simulink model "VTOL_Y4_Tiltrotor_Model"  (R2015a)
settings: Solver=ode45  StartTime=0.0  StopTime=400  RelTol=1e-3
model workspace (MAT data in the model file):
  op_trim2 : opcond.OperatingReport (value not decoded)
undefined symbols (not defined in the file): sigbuilder_block
libraries: simulink x8, aerolibutil x4, aerolibasang x2, aerolib6dof2 x1, aerolibadyn x1, aerolibconvert2 x1, aerolibtransform2 x1
settings Model: Creator=Swapneel Naphade  LastModifiedBy=HP
settings SolverCC: ZeroCrossControl=DisableAll  ZeroCrossAlgorithm=Adaptive
settings DataIOCC: ExternalInput=getinputstruct(op_trim2)  InitialState=getstatestruct(op_trim2)

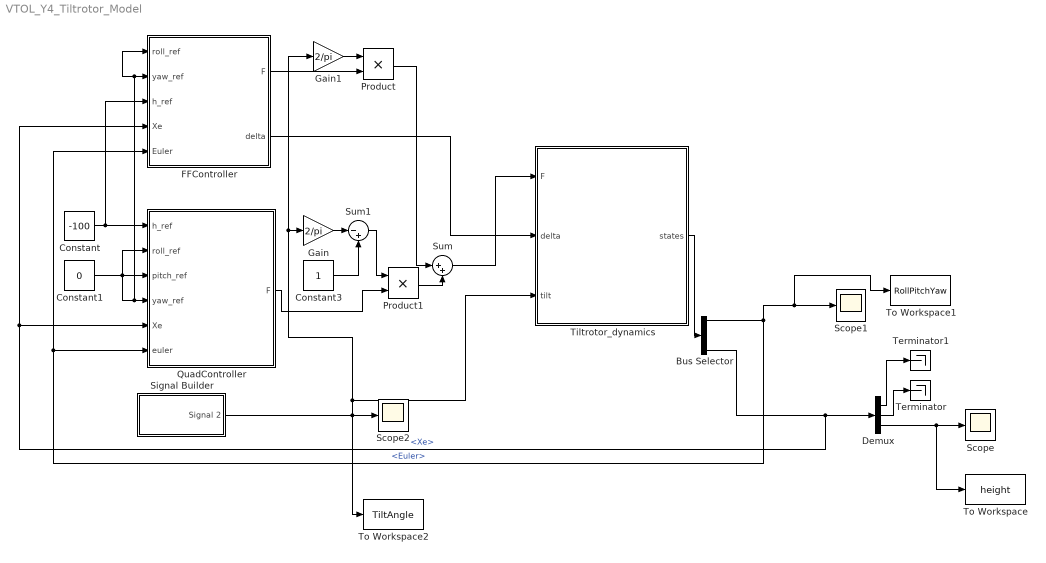
== system VTOL_Y4_Tiltrotor_Model ==
  Bus Selector : BusSelector  OutputSignals=Euler,wb,Ve,Xe
  Constant : Constant  Value=-100
  Constant1 : Constant  Value=0
  Constant3 : Constant
  Demux : Demux  Outputs=3
  FFController : Subsystem
  Gain : Gain  Gain=2/pi
  Gain1 : Gain  Gain=2/pi
  Product : Product
  Product1 : Product
  QuadController : Subsystem
  Scope : Scope
      settings: YMin=-650  YMax=-50
  Scope1 : Scope
      settings: YMin=-1.75  YMax=0.5
  Scope2 : Scope
      settings: YMin=0  YMax=1.75  SaveName=ScopeData5
  Signal Builder : Subsystem  Tag=STV Subsys  LoadFcn=sigbuilder_block('load');  StartFcn=sigbuilder_block('start');  StopFcn=sigbuilder_block('stop');  ClipboardFcn=sigbuilder_block('clipboard');  mask(Sigbuilder block){}
      mask help: Simulink:masks:SigbuilderBlock_MD
      mask init:
      | if ~strcmp(get_param(bdroot(gcbh),'SimulationStatus'),'stopped') tuvar = sigbuilder_block('maskInit'); end
      settings: CopyFcn=sigbuilder_block('copy');  DeleteFcn=sigbuilder_block('delete');  ModelCloseFcn=sigbuilder_block('modelClose');  PreSaveFcn=sigbuilder_block('preSave');  PauseFcn=sigbuilder_block('pause');  ContinueFcn=sigbuilder_block('continue');  NameChangeFcn=sigbuilder_block('namechange');  OpenFcn=sigbuilder_block('open',[437.6 199.2 550.4 400 ]);  CloseFcn=sigbuilder_block('close');
      mask Display: plot(0, 0, 100, 100,[2, 2, 32, 32, 2], [68, 8, 8, 68, 68],[32, 2], [38, 38], [32, 19, 2],[53, 60, 44], [32, 17, 17, 2],[16, 16, 31, 31]);txt = getActiveGroup(gcbh);text(2, 100, txt,'verticalAlignment', 'top');
  Sum : Sum  Inputs=|++
  Sum1 : Sum  Inputs=|-+
  Terminator : Terminator
  Terminator1 : Terminator
  Tiltrotor_dynamics : Subsystem
  To Workspace : ToWorkspace  VariableName=height  SaveFormat=Timeseries  SampleTime=-1
  To Workspace1 : ToWorkspace  VariableName=RollPitchYaw  SaveFormat=Timeseries  SampleTime=-1
  To Workspace2 : ToWorkspace  VariableName=TiltAngle  SaveFormat=Timeseries  SampleTime=-1
  wires:
  Tiltrotor_dynamics/1(states) -> Bus Selector/1
  Bus Selector/1 -> To Workspace1/1, Scope1/1, FFController/5(Euler), QuadController/6(euler)  "<Euler>"
  Bus Selector/4 -> FFController/4("Xe "), QuadController/5(Xe), Demux/1  "<Xe>"
  Demux/3 -> To Workspace/1, Scope/1
  Demux/1 -> Terminator1/1
  Demux/2 -> Terminator/1
  Constant1/1 -> FFController/1(roll_ref), FFController/2(yaw_ref), QuadController/4(yaw_ref), QuadController/2(roll_ref), QuadController/3(pitch_ref)
  FFController/2(delta) -> Tiltrotor_dynamics/2(delta)
  Constant/1 -> FFController/3(h_ref), QuadController/1(h_ref)
  QuadController/1(F) -> Product1/2
  Product1/1 -> Sum/2
  Product/1 -> Sum/1
  FFController/1(F) -> Product/2
  Sum/1 -> Tiltrotor_dynamics/1(F)
  Gain/1 -> Sum1/1
  Sum1/1 -> Product1/1
  Constant3/1 -> Sum1/2
  Gain1/1 -> Product/1
  Signal Builder/1(Signal 2) -> To Workspace2/1, Gain1/1, Gain/1, Tiltrotor_dynamics/3("tilt "), Scope2/1

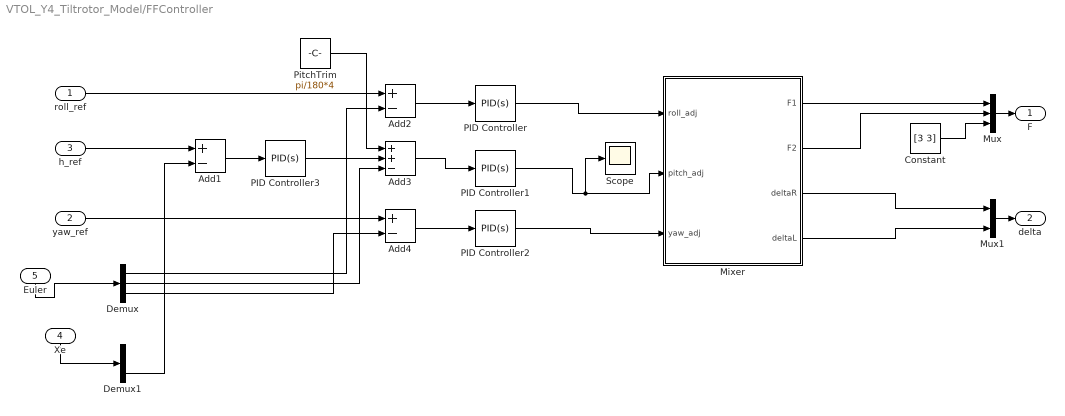
== system VTOL_Y4_Tiltrotor_Model/FFController ==
  roll_ref : Inport
  yaw_ref : Inport  Port=2
  h_ref : Inport  Port=3
  "Xe " : Inport  Port=4
  Euler : Inport  Port=5
  Add1 : Sum  Inputs=+-
  Add2 : Sum  Inputs=+-
  Add3 : Sum  Inputs=++-
  Add4 : Sum  Inputs=+-
  Constant : Constant  Value=[3 3]
  Demux : Demux  Outputs=3
  Demux1 : Demux  Outputs=3
  Mixer : Subsystem
  Mux : Mux  Inputs=3
  Mux1 : Mux  Inputs=2
  PID Controller : simulink/Continuous/PID Controller  Controller=PID  TimeDomain=Continuous-time  SampleTime=-1  IntegratorMethod=Forward Euler  FilterMethod=Forward Euler  Form=Parallel  UseFilter=on  ControllerParametersSource=internal  P=200  I=10  D=10  N=100  InitialConditionSource=internal  InitialConditionForIntegrator=0  InitialConditionForFilter=0  ExternalReset=none  LimitOutput=off  UpperSaturationLimit=inf  LowerSaturationLimit=-inf  LinearizeAsGain=on  AntiWindupMode=none  Kb=1  TrackingMode=off  Kt=1  PParamMin=[]  PParamMax=[]  IParamMin=[]  IParamMax=[]  DParamMin=[]  DParamMax=[]  NParamMin=[]  NParamMax=[]  KbParamMin=[]  KbParamMax=[]  KtParamMin=[]  KtParamMax=[]  POutMin=[]  POutMax=[]  IOutMin=[]  IOutMax=[]  DOutMin=[]  DOutMax=[]  NOutMin=[]  NOutMax=[]  KbOutMin=[]  KbOutMax=[]  KtOutMin=[]  KtOutMax=[]  IntegratorOutMin=[]  IntegratorOutMax=[]  FilterOutMin=[]  FilterOutMax=[]  SumOutMin=[]  SumOutMax=[]  SumI1OutMin=[]  SumI1OutMax=[]  SumI2OutMin=[]  SumI2OutMax=[]  SumI3OutMin=[]  SumI3OutMax=[]  SumDOutMin=[]  SumDOutMax=[]  SaturationOutMin=[]  SaturationOutMax=[]  IntegratorContinuousStateAttributes=''  IntegratorStateMustResolveToSignalObject=off  IntegratorRTWStateStorageClass=Auto  FilterContinuousStateAttributes=''  FilterStateMustResolveToSignalObject=off  FilterRTWStateStorageClass=Auto  DifferentiatorICPrevScaledInput=0  DifferentiatorOutMin=[]  DifferentiatorOutMax=[]
  PID Controller1 : simulink/Continuous/PID Controller  Controller=PID  TimeDomain=Continuous-time  SampleTime=-1  IntegratorMethod=Forward Euler  FilterMethod=Forward Euler  Form=Parallel  UseFilter=on  ControllerParametersSource=internal  P=200  I=10  D=50  N=20  InitialConditionSource=internal  InitialConditionForIntegrator=0  InitialConditionForFilter=0  ExternalReset=none  LimitOutput=off  UpperSaturationLimit=inf  LowerSaturationLimit=-inf  LinearizeAsGain=on  AntiWindupMode=none  Kb=1  TrackingMode=off  Kt=1  PParamMin=[]  PParamMax=[]  IParamMin=[]  IParamMax=[]  DParamMin=[]  DParamMax=[]  NParamMin=[]  NParamMax=[]  KbParamMin=[]  KbParamMax=[]  KtParamMin=[]  KtParamMax=[]  POutMin=[]  POutMax=[]  IOutMin=[]  IOutMax=[]  DOutMin=[]  DOutMax=[]  NOutMin=[]  NOutMax=[]  KbOutMin=[]  KbOutMax=[]  KtOutMin=[]  KtOutMax=[]  IntegratorOutMin=[]  IntegratorOutMax=[]  FilterOutMin=[]  FilterOutMax=[]  SumOutMin=[]  SumOutMax=[]  SumI1OutMin=[]  SumI1OutMax=[]  SumI2OutMin=[]  SumI2OutMax=[]  SumI3OutMin=[]  SumI3OutMax=[]  SumDOutMin=[]  SumDOutMax=[]  SaturationOutMin=[]  SaturationOutMax=[]  IntegratorContinuousStateAttributes=''  IntegratorStateMustResolveToSignalObject=off  IntegratorRTWStateStorageClass=Auto  FilterContinuousStateAttributes=''  FilterStateMustResolveToSignalObject=off  FilterRTWStateStorageClass=Auto  DifferentiatorICPrevScaledInput=0  DifferentiatorOutMin=[]  DifferentiatorOutMax=[]
  PID Controller2 : simulink/Continuous/PID Controller  Controller=PID  TimeDomain=Continuous-time  SampleTime=-1  IntegratorMethod=Forward Euler  FilterMethod=Forward Euler  Form=Parallel  UseFilter=on  ControllerParametersSource=internal  P=300  I=50  D=100  N=100  InitialConditionSource=internal  InitialConditionForIntegrator=0  InitialConditionForFilter=0  ExternalReset=none  LimitOutput=off  UpperSaturationLimit=inf  LowerSaturationLimit=-inf  LinearizeAsGain=on  AntiWindupMode=none  Kb=1  TrackingMode=off  Kt=1  PParamMin=[]  PParamMax=[]  IParamMin=[]  IParamMax=[]  DParamMin=[]  DParamMax=[]  NParamMin=[]  NParamMax=[]  KbParamMin=[]  KbParamMax=[]  KtParamMin=[]  KtParamMax=[]  POutMin=[]  POutMax=[]  IOutMin=[]  IOutMax=[]  DOutMin=[]  DOutMax=[]  NOutMin=[]  NOutMax=[]  KbOutMin=[]  KbOutMax=[]  KtOutMin=[]  KtOutMax=[]  IntegratorOutMin=[]  IntegratorOutMax=[]  FilterOutMin=[]  FilterOutMax=[]  SumOutMin=[]  SumOutMax=[]  SumI1OutMin=[]  SumI1OutMax=[]  SumI2OutMin=[]  SumI2OutMax=[]  SumI3OutMin=[]  SumI3OutMax=[]  SumDOutMin=[]  SumDOutMax=[]  SaturationOutMin=[]  SaturationOutMax=[]  IntegratorContinuousStateAttributes=''  IntegratorStateMustResolveToSignalObject=off  IntegratorRTWStateStorageClass=Auto  FilterContinuousStateAttributes=''  FilterStateMustResolveToSignalObject=off  FilterRTWStateStorageClass=Auto  DifferentiatorICPrevScaledInput=0  DifferentiatorOutMin=[]  DifferentiatorOutMax=[]
  PID Controller3 : simulink/Continuous/PID Controller  Controller=PID  TimeDomain=Continuous-time  SampleTime=-1  IntegratorMethod=Forward Euler  FilterMethod=Forward Euler  Form=Parallel  UseFilter=on  ControllerParametersSource=internal  P=-.05  I=-.001  D=-.001  N=20  InitialConditionSource=internal  InitialConditionForIntegrator=0  InitialConditionForFilter=0  ExternalReset=none  LimitOutput=off  UpperSaturationLimit=inf  LowerSaturationLimit=-inf  LinearizeAsGain=on  AntiWindupMode=none  Kb=1  TrackingMode=off  Kt=1  PParamMin=[]  PParamMax=[]  IParamMin=[]  IParamMax=[]  DParamMin=[]  DParamMax=[]  NParamMin=[]  NParamMax=[]  KbParamMin=[]  KbParamMax=[]  KtParamMin=[]  KtParamMax=[]  POutMin=[]  POutMax=[]  IOutMin=[]  IOutMax=[]  DOutMin=[]  DOutMax=[]  NOutMin=[]  NOutMax=[]  KbOutMin=[]  KbOutMax=[]  KtOutMin=[]  KtOutMax=[]  IntegratorOutMin=[]  IntegratorOutMax=[]  FilterOutMin=[]  FilterOutMax=[]  SumOutMin=[]  SumOutMax=[]  SumI1OutMin=[]  SumI1OutMax=[]  SumI2OutMin=[]  SumI2OutMax=[]  SumI3OutMin=[]  SumI3OutMax=[]  SumDOutMin=[]  SumDOutMax=[]  SaturationOutMin=[]  SaturationOutMax=[]  IntegratorContinuousStateAttributes=''  IntegratorStateMustResolveToSignalObject=off  IntegratorRTWStateStorageClass=Auto  FilterContinuousStateAttributes=''  FilterStateMustResolveToSignalObject=off  FilterRTWStateStorageClass=Auto  DifferentiatorICPrevScaledInput=0  DifferentiatorOutMin=[]  DifferentiatorOutMax=[]
  PitchTrim : Constant  Value=pi/180*4
  Scope : Scope
      settings: YMin=-1e+06  YMax=50000  SaveName=ScopeData3
  F : Outport
  delta : Outport  Port=2
  wires:
  Euler/1 -> Demux/1
  Mixer/1(F1) -> Mux/1
  PID Controller2/1 -> Mixer/3(yaw_adj)
  PID Controller/1 -> Mixer/1(roll_adj)
  Mixer/2(F2) -> Mux/2
  PID Controller1/1 -> Scope/1, Mixer/2(pitch_adj)
  Add2/1 -> PID Controller/1
  Demux/1 -> Add2/2
  Add4/1 -> PID Controller2/1
  Add3/1 -> PID Controller1/1
  Demux/2 -> Add3/3
  roll_ref/1 -> Add2/1
  Demux/3 -> Add4/2
  h_ref/1 -> Add1/1
  PID Controller3/1 -> Add3/2
  Add1/1 -> PID Controller3/1
  "Xe "/1 -> Demux1/1
  Demux1/3 -> Add1/2
  yaw_ref/1 -> Add4/1
  Constant/1 -> Mux/3
  Mux/1 -> F/1
  Mixer/3(deltaR) -> Mux1/1
  Mixer/4(deltaL) -> Mux1/2
  Mux1/1 -> delta/1
  PitchTrim/1 -> Add3/1

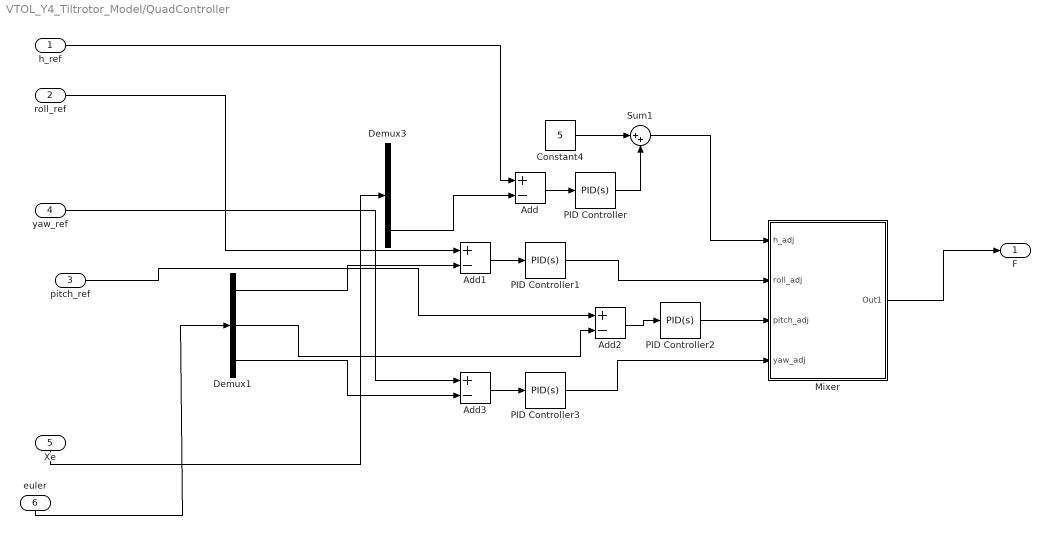
== system VTOL_Y4_Tiltrotor_Model/QuadController ==
  h_ref : Inport
  roll_ref : Inport  Port=2
  pitch_ref : Inport  Port=3
  yaw_ref : Inport  Port=4
  Xe : Inport  Port=5
  euler : Inport  Port=6
  Add{,1..3} (4 alike) : Sum  Inputs=+-
  Constant4 : Constant  Value=5
  Demux1 : Demux  Outputs=3
  Demux3 : Demux  Outputs=3
  Mixer : Subsystem
  PID Controller : simulink/Continuous/PID Controller  Controller=PID  TimeDomain=Continuous-time  SampleTime=-1  IntegratorMethod=Forward Euler  FilterMethod=Forward Euler  Form=Parallel  UseFilter=off  ControllerParametersSource=internal  P=-50  I=0  D=-100  N=100  InitialConditionSource=internal  InitialConditionForIntegrator=0  InitialConditionForFilter=0  ExternalReset=none  LimitOutput=off  UpperSaturationLimit=inf  LowerSaturationLimit=-inf  LinearizeAsGain=on  AntiWindupMode=none  Kb=1  TrackingMode=off  Kt=1  PParamMin=[]  PParamMax=[]  IParamMin=[]  IParamMax=[]  DParamMin=[]  DParamMax=[]  NParamMin=[]  NParamMax=[]  KbParamMin=[]  KbParamMax=[]  KtParamMin=[]  KtParamMax=[]  POutMin=[]  POutMax=[]  IOutMin=[]  IOutMax=[]  DOutMin=[]  DOutMax=[]  NOutMin=[]  NOutMax=[]  KbOutMin=[]  KbOutMax=[]  KtOutMin=[]  KtOutMax=[]  IntegratorOutMin=[]  IntegratorOutMax=[]  FilterOutMin=[]  FilterOutMax=[]  SumOutMin=[]  SumOutMax=[]  SumI1OutMin=[]  SumI1OutMax=[]  SumI2OutMin=[]  SumI2OutMax=[]  SumI3OutMin=[]  SumI3OutMax=[]  SumDOutMin=[]  SumDOutMax=[]  SaturationOutMin=[]  SaturationOutMax=[]  IntegratorContinuousStateAttributes=''  IntegratorStateMustResolveToSignalObject=off  IntegratorRTWStateStorageClass=Auto  FilterContinuousStateAttributes=''  FilterStateMustResolveToSignalObject=off  FilterRTWStateStorageClass=Auto  DifferentiatorICPrevScaledInput=0  DifferentiatorOutMin=[]  DifferentiatorOutMax=[]
  PID Controller1 : simulink/Continuous/PID Controller  Controller=PID  TimeDomain=Continuous-time  SampleTime=-1  IntegratorMethod=Forward Euler  FilterMethod=Forward Euler  Form=Parallel  UseFilter=on  ControllerParametersSource=internal  P=50  I=1  D=50  N=100  InitialConditionSource=internal  InitialConditionForIntegrator=0  InitialConditionForFilter=0  ExternalReset=none  LimitOutput=off  UpperSaturationLimit=inf  LowerSaturationLimit=-inf  LinearizeAsGain=on  AntiWindupMode=none  Kb=1  TrackingMode=off  Kt=1  PParamMin=[]  PParamMax=[]  IParamMin=[]  IParamMax=[]  DParamMin=[]  DParamMax=[]  NParamMin=[]  NParamMax=[]  KbParamMin=[]  KbParamMax=[]  KtParamMin=[]  KtParamMax=[]  POutMin=[]  POutMax=[]  IOutMin=[]  IOutMax=[]  DOutMin=[]  DOutMax=[]  NOutMin=[]  NOutMax=[]  KbOutMin=[]  KbOutMax=[]  KtOutMin=[]  KtOutMax=[]  IntegratorOutMin=[]  IntegratorOutMax=[]  FilterOutMin=[]  FilterOutMax=[]  SumOutMin=[]  SumOutMax=[]  SumI1OutMin=[]  SumI1OutMax=[]  SumI2OutMin=[]  SumI2OutMax=[]  SumI3OutMin=[]  SumI3OutMax=[]  SumDOutMin=[]  SumDOutMax=[]  SaturationOutMin=[]  SaturationOutMax=[]  IntegratorContinuousStateAttributes=''  IntegratorStateMustResolveToSignalObject=off  IntegratorRTWStateStorageClass=Auto  FilterContinuousStateAttributes=''  FilterStateMustResolveToSignalObject=off  FilterRTWStateStorageClass=Auto  DifferentiatorICPrevScaledInput=0  DifferentiatorOutMin=[]  DifferentiatorOutMax=[]
  PID Controller2 : simulink/Continuous/PID Controller  Controller=PID  TimeDomain=Continuous-time  SampleTime=-1  IntegratorMethod=Forward Euler  FilterMethod=Forward Euler  Form=Parallel  UseFilter=on  ControllerParametersSource=internal  P=300  I=10  D=100  N=100  InitialConditionSource=internal  InitialConditionForIntegrator=0  InitialConditionForFilter=0  ExternalReset=none  LimitOutput=off  UpperSaturationLimit=inf  LowerSaturationLimit=-inf  LinearizeAsGain=on  AntiWindupMode=none  Kb=1  TrackingMode=off  Kt=1  PParamMin=[]  PParamMax=[]  IParamMin=[]  IParamMax=[]  DParamMin=[]  DParamMax=[]  NParamMin=[]  NParamMax=[]  KbParamMin=[]  KbParamMax=[]  KtParamMin=[]  KtParamMax=[]  POutMin=[]  POutMax=[]  IOutMin=[]  IOutMax=[]  DOutMin=[]  DOutMax=[]  NOutMin=[]  NOutMax=[]  KbOutMin=[]  KbOutMax=[]  KtOutMin=[]  KtOutMax=[]  IntegratorOutMin=[]  IntegratorOutMax=[]  FilterOutMin=[]  FilterOutMax=[]  SumOutMin=[]  SumOutMax=[]  SumI1OutMin=[]  SumI1OutMax=[]  SumI2OutMin=[]  SumI2OutMax=[]  SumI3OutMin=[]  SumI3OutMax=[]  SumDOutMin=[]  SumDOutMax=[]  SaturationOutMin=[]  SaturationOutMax=[]  IntegratorContinuousStateAttributes=''  IntegratorStateMustResolveToSignalObject=off  IntegratorRTWStateStorageClass=Auto  FilterContinuousStateAttributes=''  FilterStateMustResolveToSignalObject=off  FilterRTWStateStorageClass=Auto  DifferentiatorICPrevScaledInput=0  DifferentiatorOutMin=[]  DifferentiatorOutMax=[]
  PID Controller3 : simulink/Continuous/PID Controller  Controller=PID  TimeDomain=Continuous-time  SampleTime=-1  IntegratorMethod=Forward Euler  FilterMethod=Forward Euler  Form=Parallel  UseFilter=on  ControllerParametersSource=internal  P=-200  I=1  D=-10  N=100  InitialConditionSource=internal  InitialConditionForIntegrator=0  InitialConditionForFilter=0  ExternalReset=none  LimitOutput=off  UpperSaturationLimit=inf  LowerSaturationLimit=-inf  LinearizeAsGain=on  AntiWindupMode=none  Kb=1  TrackingMode=off  Kt=1  PParamMin=[]  PParamMax=[]  IParamMin=[]  IParamMax=[]  DParamMin=[]  DParamMax=[]  NParamMin=[]  NParamMax=[]  KbParamMin=[]  KbParamMax=[]  KtParamMin=[]  KtParamMax=[]  POutMin=[]  POutMax=[]  IOutMin=[]  IOutMax=[]  DOutMin=[]  DOutMax=[]  NOutMin=[]  NOutMax=[]  KbOutMin=[]  KbOutMax=[]  KtOutMin=[]  KtOutMax=[]  IntegratorOutMin=[]  IntegratorOutMax=[]  FilterOutMin=[]  FilterOutMax=[]  SumOutMin=[]  SumOutMax=[]  SumI1OutMin=[]  SumI1OutMax=[]  SumI2OutMin=[]  SumI2OutMax=[]  SumI3OutMin=[]  SumI3OutMax=[]  SumDOutMin=[]  SumDOutMax=[]  SaturationOutMin=[]  SaturationOutMax=[]  IntegratorContinuousStateAttributes=''  IntegratorStateMustResolveToSignalObject=off  IntegratorRTWStateStorageClass=Auto  FilterContinuousStateAttributes=''  FilterStateMustResolveToSignalObject=off  FilterRTWStateStorageClass=Auto  DifferentiatorICPrevScaledInput=0  DifferentiatorOutMin=[]  DifferentiatorOutMax=[]
  Sum1 : Sum  Inputs=|++
  F : Outport
  wires:
  Demux3/3 -> Add/2
  Add2/1 -> PID Controller2/1
  Add3/1 -> PID Controller3/1
  Demux1/1 -> Add1/2
  PID Controller/1 -> Sum1/2
  Add/1 -> PID Controller/1
  h_ref/1 -> Add/1
  yaw_ref/1 -> Add3/1
  Sum1/1 -> Mixer/1(h_adj)
  Add1/1 -> PID Controller1/1
  PID Controller1/1 -> Mixer/2(roll_adj)
  PID Controller3/1 -> Mixer/4(yaw_adj)
  Demux1/3 -> Add3/2
  Constant4/1 -> Sum1/1
  Mixer/1(Out1) -> F/1
  PID Controller2/1 -> Mixer/3(pitch_adj)
  roll_ref/1 -> Add1/1
  euler/1 -> Demux1/1
  Xe/1 -> Demux3/1
  Demux1/2 -> Add2/2
  pitch_ref/1 -> Add2/1

== system VTOL_Y4_Tiltrotor_Model/Signal Builder ==
  Demux : Demux  Tag=STV Demux  Outputs=1
  FromWs : FromWorkspace  Tag=STV FromWs  VariableName=tuvar  SampleTime=0
      SigBuilderData=|
      | common.afterFinalStr = 'Extrapolate'
      | common.sampleTime = 0
      | dataSet.timeRange = [0 400]
      | dataSet.name = 'Group 1'
      | sbobj.Groups.Name = 'Group 1'
      | sbobj.Groups.Signals.Name = 'Signal 2'
      | sbobj.Groups.Signals.XData = [0 40 60 230 260 400]
      | sbobj.Groups.Signals.YData = [0 0 1.57079632679 1.57079632679 0 0]
      | sbobj.Groups.TimeRange = [0 400]
  Signal 2 : Outport  Tag=STV Outport
  wires:
  FromWs/1 -> Demux/1
  Demux/1 -> Signal 2/1

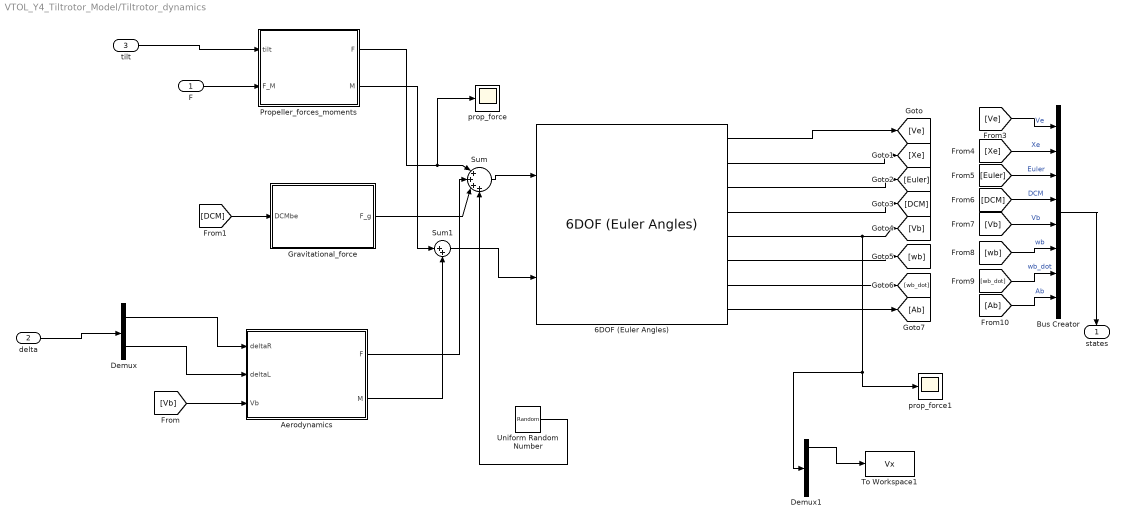
== system VTOL_Y4_Tiltrotor_Model/Tiltrotor_dynamics ==
  F : Inport
  delta : Inport  Port=2
  "tilt " : Inport  Port=3
  6DOF (Euler Angles) : aerolib6dof2/6DOF (Euler Angles)  units=Metric (MKS)  mtype=Fixed  rep=Euler Angles  xme_0=[0 0 -100]  Vm_0=[0 0 0]  eul_0=[0 0 0]  pm_0=[0 0 0]  mass_0=5  mass_e=0.5  mass_f=2.0  inertia=[1 0 0; 0 1 0; 0 0 1]  inertia_e=eye(3)  inertia_f=2*eye(3)  k_quat=1.0  vre_flag=on
  Aerodynamics : Subsystem
  Bus Creator : BusCreator  Inputs='Ve','Xe','Euler','DCM','Vb','wb','wb_dot','Ab'
  Demux : Demux  Outputs=2
  Demux1 : Demux  Outputs=3
  Gravitational_force : Subsystem
  Propeller_forces_moments : Subsystem
  Sum : Sum  Inputs=|++++
  Sum1 : Sum  Inputs=|++
  To Workspace1 : ToWorkspace  VariableName=Vx  SaveFormat=Timeseries  SampleTime=-1
  Uniform Random Number : UniformRandomNumber  Minimum=2*[-1 -1 -1]  Maximum=2*[1 1 1]  SampleTime=0.1
  prop_force : Scope
      settings: YMin=0  YMax=175  SaveName=ScopeData4
  prop_force1 : Scope
      settings: YMin=-450  YMax=400  SaveName=ScopeData2
  states : Outport
  wires:
  Propeller_forces_moments/1(F) -> prop_force/1, Sum/1
  6DOF (Euler Angles)/1 -> [Ve]
  6DOF (Euler Angles)/5 -> Demux1/1, prop_force1/1, [Vb]
  Sum1/1 -> 6DOF (Euler Angles)/2
  Propeller_forces_moments/2(M) -> Sum1/1
  6DOF (Euler Angles)/3 -> [Euler]
  6DOF (Euler Angles)/8 -> [Ab]
  6DOF (Euler Angles)/6 -> [wb]
  6DOF (Euler Angles)/7 -> [wb_dot]
  6DOF (Euler Angles)/4 -> [DCM]
  Sum/1 -> 6DOF (Euler Angles)/1
  Gravitational_force/1(F_g) -> Sum/3
  "tilt "/1 -> Propeller_forces_moments/1(tilt)
  [Vb] -> Aerodynamics/3("Vb ")
  [Ve] -> Bus Creator/1  "Ve"
  Bus Creator/1 -> states/1
  [DCM] -> Gravitational_force/1(DCMbe)
  [Ab] -> Bus Creator/8  "Ab"
  [Xe] -> Bus Creator/2  "Xe"
  [DCM] -> Bus Creator/4  "DCM"
  [wb_dot] -> Bus Creator/7  "wb_dot"
  [Euler] -> Bus Creator/3  "Euler"
  [wb] -> Bus Creator/6  "wb"
  F/1 -> Propeller_forces_moments/2(F_M)
  [Vb] -> Bus Creator/5  "Vb"
  6DOF (Euler Angles)/2 -> [Xe]
  Demux/2 -> Aerodynamics/2(deltaL)
  delta/1 -> Demux/1
  Demux/1 -> Aerodynamics/1(deltaR)
  Aerodynamics/1(F) -> Sum/2
  Aerodynamics/2(M) -> Sum1/2
  Uniform Random Number/1 -> Sum/4
  Demux1/1 -> To Workspace1/1

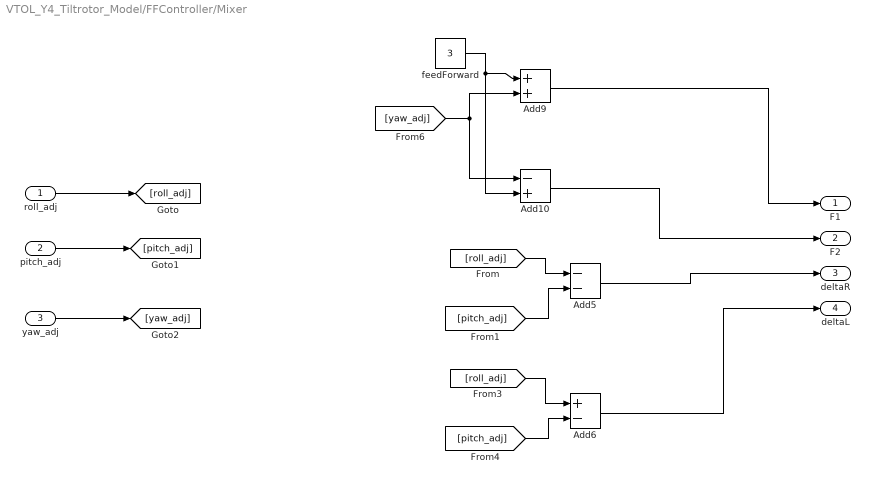
== system VTOL_Y4_Tiltrotor_Model/FFController/Mixer ==
  roll_adj : Inport
  pitch_adj : Inport  Port=2
  yaw_adj : Inport  Port=3
  Add10 : Sum  Inputs=-+
  Add5 : Sum  Inputs=--
  Add6 : Sum  Inputs=+-
  Add9 : Sum
  feedForward : Constant  Value=3
  F1 : Outport
  F2 : Outport  Port=2
  deltaR : Outport  Port=3
  deltaL : Outport  Port=4
  wires:
  Add5/1 -> deltaR/1
  Add9/1 -> F1/1
  roll_adj/1 -> [roll_adj]
  pitch_adj/1 -> [pitch_adj]
  [roll_adj] -> Add6/1
  [pitch_adj] -> Add5/2
  yaw_adj/1 -> [yaw_adj]
  [roll_adj] -> Add5/1
  [pitch_adj] -> Add6/2
  [yaw_adj] -> Add9/2, Add10/1
  Add10/1 -> F2/1
  Add6/1 -> deltaL/1
  feedForward/1 -> Add10/2, Add9/1

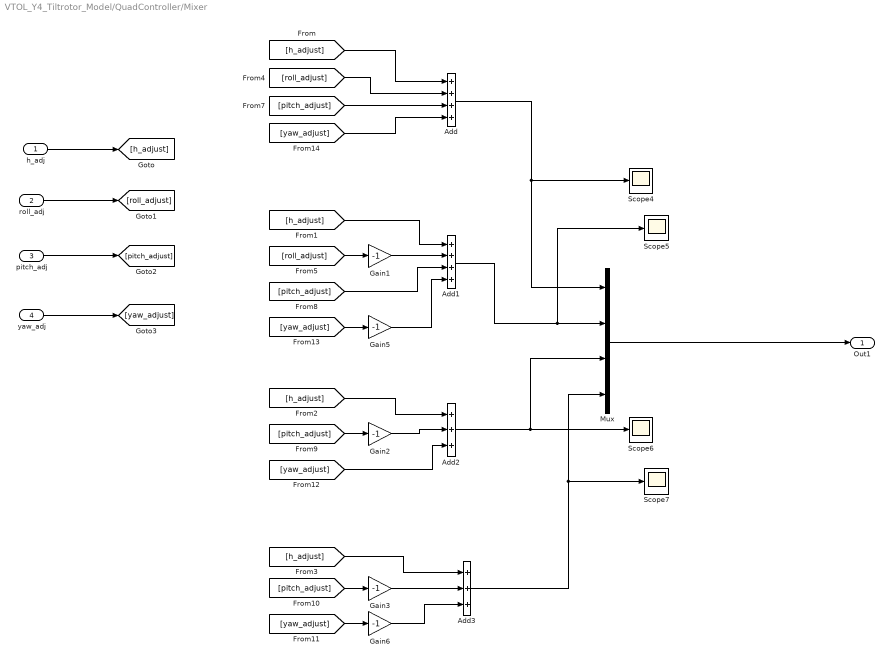
== system VTOL_Y4_Tiltrotor_Model/QuadController/Mixer ==
  h_adj : Inport
  roll_adj : Inport  Port=2
  pitch_adj : Inport  Port=3
  yaw_adj : Inport  Port=4
  Add : Sum  Inputs=++++
  Add1 : Sum  Inputs=++++
  Add2 : Sum  Inputs=+++
  Add3 : Sum  Inputs=+++
  Gain{1..3,5..6} (5 alike) : Gain  Gain=-1
  Mux : Mux
  Scope{4..7} (4 alike) : Scope
      Scope4 settings: ShowLegends=on  YMin=-1.2e+06  YMax=0  SaveName=ScopeData11  ScrollMode=on
      Scope5 settings: ShowLegends=on  YMin=0  YMax=19000  SaveName=ScopeData12  ScrollMode=on
      Scope6 settings: ShowLegends=on  YMin=-45000  YMax=5000  SaveName=ScopeData13  ScrollMode=on
      Scope7 settings: ShowLegends=on  YMax=100  SaveName=ScopeData14  ScrollMode=on
  Out1 : Outport
  wires:
  yaw_adj/1 -> [yaw_adjust]
  roll_adj/1 -> [roll_adjust]
  pitch_adj/1 -> [pitch_adjust]
  [roll_adjust] -> Gain1/1
  [pitch_adjust] -> Gain3/1
  [h_adjust] -> Add/1
  [yaw_adjust] -> Gain5/1
  Gain3/1 -> Add3/2
  [h_adjust] -> Add2/1
  [pitch_adjust] -> Add1/3
  Add/1 -> Mux/1, Scope4/1
  Add1/1 -> Scope5/1, Mux/2
  Gain5/1 -> Add1/4
  Gain1/1 -> Add1/2
  Gain2/1 -> Add2/2
  [roll_adjust] -> Add/2
  [pitch_adjust] -> Add/3
  [yaw_adjust] -> Add2/3
  Add2/1 -> Mux/3, Scope6/1
  [yaw_adjust] -> Gain6/1
  Add3/1 -> Mux/4, Scope7/1
  [h_adjust] -> Add3/1
  [h_adjust] -> Add1/1
  Mux/1 -> Out1/1
  [pitch_adjust] -> Gain2/1
  h_adj/1 -> [h_adjust]
  [yaw_adjust] -> Add/4
  Gain6/1 -> Add3/3

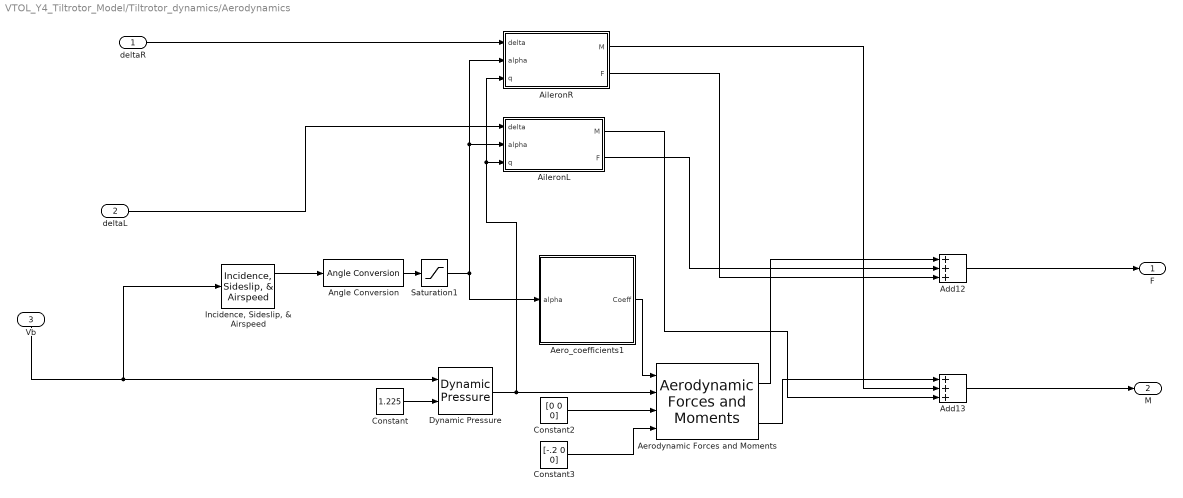
== system VTOL_Y4_Tiltrotor_Model/Tiltrotor_dynamics/Aerodynamics ==
  deltaR : Inport
  deltaL : Inport  Port=2
  "Vb " : Inport  Port=3
  Add12 : Sum  Inputs=+++
  Add13 : Sum  Inputs=+++
  Aero_coefficients1 : Subsystem
  "Aerodynamic Forces and Moments " : aerolibadyn/Aerodynamic Forces and Moments   inputAxes=Body  outputForceAxes=Body  outputMomentAxes=Body  S=1.02  b=2.11  cbar=.492
  AileronL : Subsystem
  AileronR : Subsystem
  Angle Conversion : aerolibconvert2/Angle Conversion  IU=rad  OU=deg
  Constant : Constant  Value=1.225
  Constant2 : Constant  Value=[0 0 0]
  Constant3 : Constant  Value=[-.2 0 0]
  Dynamic Pressure : aerolibasang/Dynamic Pressure
  "Incidence, Sideslip, & Airspeed" : aerolibasang/Incidence, Sideslip, & Airspeed
  Saturation1 : Saturate  UpperLimit=20  LowerLimit=-20
  F : Outport
  M : Outport  Port=2
  wires:
  AileronR/2(F) -> Add12/3
  AileronL/1(M) -> Add13/3
  Add12/1 -> F/1
  AileronL/2(F) -> Add12/2
  "Aerodynamic Forces and Moments "/1 -> Add12/1
  AileronR/1(M) -> Add13/2
  "Aerodynamic Forces and Moments "/2 -> Add13/1
  Add13/1 -> M/1
  Angle Conversion/1 -> Saturation1/1
  Constant3/1 -> "Aerodynamic Forces and Moments "/4
  Aero_coefficients1/1(Coeff) -> "Aerodynamic Forces and Moments "/1
  "Incidence, Sideslip, & Airspeed"/1 -> Angle Conversion/1
  Constant2/1 -> "Aerodynamic Forces and Moments "/3
  Dynamic Pressure/1 -> AileronR/3(q), AileronL/3(q), "Aerodynamic Forces and Moments "/2
  Constant/1 -> Dynamic Pressure/2
  Saturation1/1 -> Aero_coefficients1/1(alpha), AileronR/2(alpha), AileronL/2(alpha)
  deltaL/1 -> AileronL/1(delta)
  deltaR/1 -> AileronR/1(delta)
  "Vb "/1 -> Dynamic Pressure/1, "Incidence, Sideslip, & Airspeed"/1

== system VTOL_Y4_Tiltrotor_Model/Tiltrotor_dynamics/Gravitational_force ==
  DCMbe : Inport
  Constant1 : Constant  Value=[0; 0; 9.81]
  Product1 : Product  Multiplication=Matrix(*)
  mass : Gain  Gain=5
  F_g : Outport
  wires:
  Constant1/1 -> mass/1
  DCMbe/1 -> Product1/1
  mass/1 -> Product1/2
  Product1/1 -> F_g/1

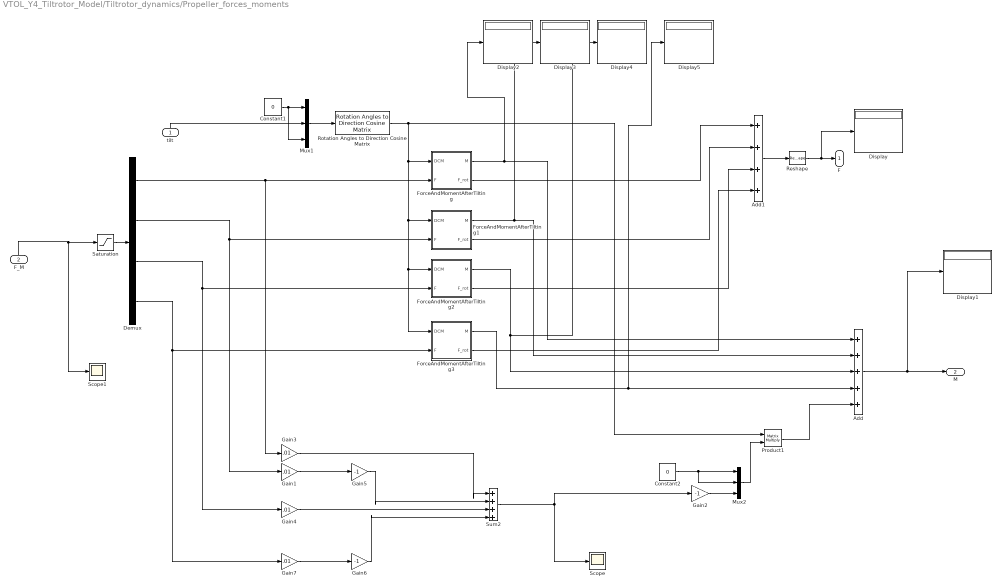
== system VTOL_Y4_Tiltrotor_Model/Tiltrotor_dynamics/Propeller_forces_moments ==
  tilt : Inport
  F_M : Inport  Port=2
  Add : Sum  Inputs=+++++
  Add1 : Sum  Inputs=++++
  Constant1 : Constant  Value=0
  Constant2 : Constant  Value=0
  Demux : Demux
  Display{,1..5} (6 alike) : Display
  ForceAndMomentAfterTilting : Subsystem
  ForceAndMomentAfterTilting1 : Subsystem
  ForceAndMomentAfterTilting2 : Subsystem
  ForceAndMomentAfterTilting3 : Subsystem
  Gain{1,3..4,7} (4 alike) : Gain  Gain=.01
  Gain2 : Gain  Gain=-1
  Gain5 : Gain  Gain=-1
  Gain6 : Gain  Gain=-1
  Mux1 : Mux  Inputs=3
  Mux2 : Mux  Inputs=3
  Product1 : Product  Multiplication=Matrix(*)
  Reshape : Reshape
  Rotation Angles to Direction Cosine Matrix : aerolibtransform2/Rotation Angles to Direction Cosine Matrix  rotationOrder=ZYX
  Saturation : Saturate  UpperLimit=50  LowerLimit=0
  Scope : Scope
      settings: YMin=-3.475e+09  YMax=-3.275e+09  SaveName=ScopeData9
  Scope1 : Scope
      settings: YMin=-900000  YMax=1.1e+06  SaveName=ScopeData10
  Sum2 : Sum  Inputs=|++++
  F : Outport
  M : Outport  Port=2
  wires:
  Mux1/1 -> Rotation Angles to Direction Cosine Matrix/1
  F_M/1 -> Saturation/1, Scope1/1
  Add1/1 -> Reshape/1
  Rotation Angles to Direction Cosine Matrix/1 -> ForceAndMomentAfterTilting1/1(DCM), ForceAndMomentAfterTilting3/1(DCM), ForceAndMomentAfterTilting2/1(DCM), ForceAndMomentAfterTilting/1(DCM), Product1/1
  Constant1/1 -> Mux1/1, Mux1/3
  Demux/4 -> Gain7/1, ForceAndMomentAfterTilting3/2(F)
  tilt/1 -> Mux1/2
  Mux2/1 -> Product1/2
  Gain2/1 -> Mux2/3
  Sum2/1 -> Scope/1, Gain2/1
  Demux/2 -> Gain1/1, ForceAndMomentAfterTilting1/2(F)
  Demux/3 -> Gain4/1, ForceAndMomentAfterTilting2/2(F)
  Constant2/1 -> Mux2/1, Mux2/2
  Product1/1 -> Add/5
  ForceAndMomentAfterTilting/1(M) -> Display2/1, Add/1
  ForceAndMomentAfterTilting1/1(M) -> Display3/1, Add/2
  ForceAndMomentAfterTilting2/1(M) -> Display4/1, Add/3
  ForceAndMomentAfterTilting3/1(M) -> Display5/1, Add/4
  Add/1 -> Display1/1, M/1
  ForceAndMomentAfterTilting/2(F_rot) -> Add1/1
  ForceAndMomentAfterTilting1/2(F_rot) -> Add1/2
  ForceAndMomentAfterTilting2/2(F_rot) -> Add1/3
  ForceAndMomentAfterTilting3/2(F_rot) -> Add1/4
  Demux/1 -> ForceAndMomentAfterTilting/2(F), Gain3/1
  Gain5/1 -> Sum2/2
  Gain6/1 -> Sum2/4
  Saturation/1 -> Demux/1
  Reshape/1 -> F/1, Display/1
  Gain1/1 -> Gain5/1
  Gain3/1 -> Sum2/1
  Gain4/1 -> Sum2/3
  Gain7/1 -> Gain6/1

== system VTOL_Y4_Tiltrotor_Model/Tiltrotor_dynamics/Aerodynamics/Aero_coefficients1 ==
  alpha : Inport
  CD : Lookup_n-D  NumberOfTableDimensions=1  BreakpointsForDimension1=[-20:20]  Table=-.0002*([-20:20]).^2-.001  InternalRulePriority=Speed  RndMeth=Simplest  InputSameDT=on
  CL : Lookup_n-D  NumberOfTableDimensions=1  BreakpointsForDimension1=[-20:20]  Table=-.0485*([-20:20])-.0067  InternalRulePriority=Speed  RndMeth=Simplest  InputSameDT=on
  Cl : Constant  Value=0
  Cm : Lookup_n-D  NumberOfTableDimensions=1  BreakpointsForDimension1=[-20:20]  Table=-.003*([-20:20])-.0015  InternalRulePriority=Speed  RndMeth=Simplest  InputSameDT=on
  Mux : Mux  Inputs=6
  Coeff : Outport
  wires:
  alpha/1 -> Cm/1, CL/1, CD/1
  Mux/1 -> Coeff/1
  CD/1 -> Mux/1
  Cm/1 -> Mux/5
  CL/1 -> Mux/3
  Cl/1 -> Mux/2, Mux/6, Mux/4

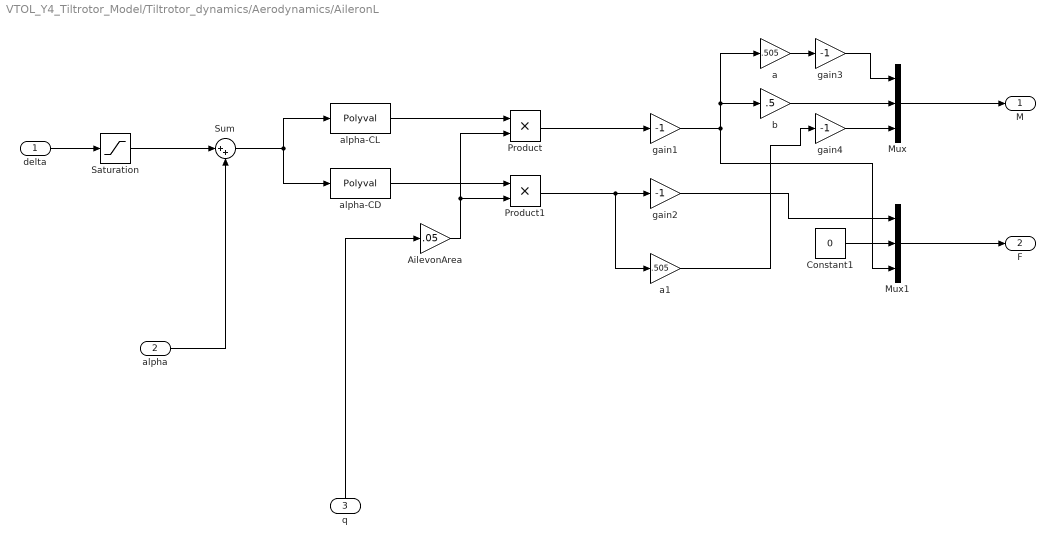
== system VTOL_Y4_Tiltrotor_Model/Tiltrotor_dynamics/Aerodynamics/AileronL ==
  delta : Inport
  alpha : Inport  Port=2
  q : Inport  Port=3
  AilevonArea : Gain  Gain=.05
  Constant1 : Constant  Value=0
  Mux : Mux  Inputs=3
  Mux1 : Mux  Inputs=3
  Product : Product
  Product1 : Product
  Saturation : Saturate  UpperLimit=10  LowerLimit=-10
  Sum : Sum  Inputs=|++
  a : Gain  Gain=.505
  a1 : Gain  Gain=.505
  alpha-CD : Polyval  Coefs=[2e-5 2e-8 -5e-5 -4e-7 .0119]
  alpha-CL : Polyval  Coefs=[0.0987 0]
  b : Gain  Gain=.5
  gain{1..4} (4 alike) : Gain  Gain=-1
  M : Outport
  F : Outport  Port=2
  wires:
  gain1/1 -> b/1, a/1, Mux1/3
  Product1/1 -> gain2/1, a1/1
  delta/1 -> Saturation/1
  AilevonArea/1 -> Product1/2, Product/2
  Sum/1 -> alpha-CL/1, alpha-CD/1
  b/1 -> Mux/2
  gain2/1 -> Mux1/1
  Mux1/1 -> F/1
  a1/1 -> gain4/1
  Product/1 -> gain1/1
  Constant1/1 -> Mux1/2
  Mux/1 -> M/1
  alpha-CL/1 -> Product/1
  alpha-CD/1 -> Product1/1
  alpha/1 -> Sum/2
  q/1 -> AilevonArea/1
  a/1 -> gain3/1
  gain3/1 -> Mux/1
  gain4/1 -> Mux/3
  Saturation/1 -> Sum/1

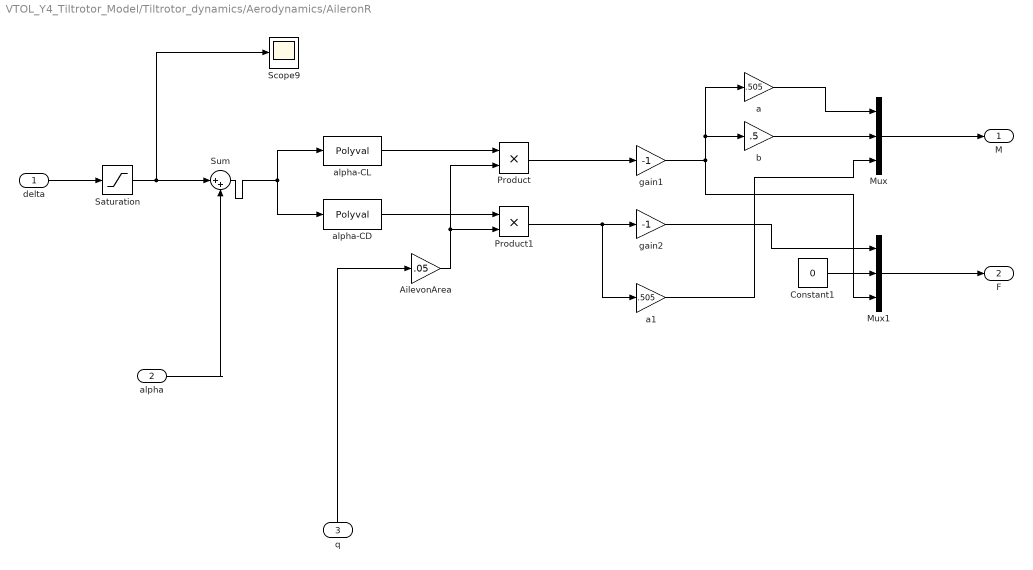
== system VTOL_Y4_Tiltrotor_Model/Tiltrotor_dynamics/Aerodynamics/AileronR ==
  delta : Inport
  alpha : Inport  Port=2
  q : Inport  Port=3
  AilevonArea : Gain  Gain=.05
  Constant1 : Constant  Value=0
  Mux : Mux  Inputs=3
  Mux1 : Mux  Inputs=3
  Product : Product
  Product1 : Product
  Saturation : Saturate  UpperLimit=10  LowerLimit=-10
  Scope9 : Scope
      settings: YMin=-20  YMax=-20  SaveName=ScopeData9
  Sum : Sum  Inputs=|++
  a : Gain  Gain=.505
  a1 : Gain  Gain=.505
  alpha-CD : Polyval  Coefs=[2e-5 2e-8 -5e-5 -4e-7 0]
  alpha-CL : Polyval  Coefs=[0.0987 0]
  b : Gain  Gain=.5
  gain1 : Gain  Gain=-1
  gain2 : Gain  Gain=-1
  M : Outport
  F : Outport  Port=2
  wires:
  q/1 -> AilevonArea/1
  alpha/1 -> Sum/2
  a/1 -> Mux/1
  alpha-CD/1 -> Product1/1
  alpha-CL/1 -> Product/1
  Mux/1 -> M/1
  Constant1/1 -> Mux1/2
  Product/1 -> gain1/1
  a1/1 -> Mux/3
  Mux1/1 -> F/1
  gain2/1 -> Mux1/1
  b/1 -> Mux/2
  Sum/1 -> alpha-CD/1, alpha-CL/1
  AilevonArea/1 -> Product/2, Product1/2
  delta/1 -> Saturation/1
  Product1/1 -> a1/1, gain2/1
  gain1/1 -> Mux1/3, a/1, b/1
  Saturation/1 -> Scope9/1, Sum/1

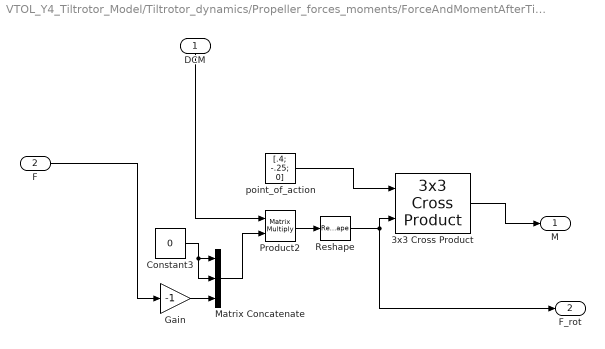
== system VTOL_Y4_Tiltrotor_Model/Tiltrotor_dynamics/Propeller_forces_moments/ForceAndMomentAfterTilting ==
  DCM : Inport
  F : Inport  Port=2
  3x3 Cross Product : aerolibutil/3x3 Cross Product
  Constant3 : Constant  Value=0
  Gain : Gain  Gain=-1
  Matrix Concatenate : Concatenate  NumInputs=3  ConcatenateDimension=2
  Product2 : Product  Multiplication=Matrix(*)
  Reshape : Reshape  OutputDimensionality=Customize  OutputDimensions=[3,1]
  point_of_action : Constant  Value="[.4;  -.25;  0]"  VectorParams1D=off
  M : Outport
  F_rot : Outport  Port=2
  wires:
  3x3 Cross Product/1 -> M/1
  F/1 -> Gain/1
  DCM/1 -> Product2/1
  Matrix Concatenate/1 -> Product2/2
  Constant3/1 -> Matrix Concatenate/2, Matrix Concatenate/1
  point_of_action/1 -> 3x3 Cross Product/1
  Product2/1 -> Reshape/1
  Reshape/1 -> 3x3 Cross Product/2, F_rot/1
  Gain/1 -> Matrix Concatenate/3

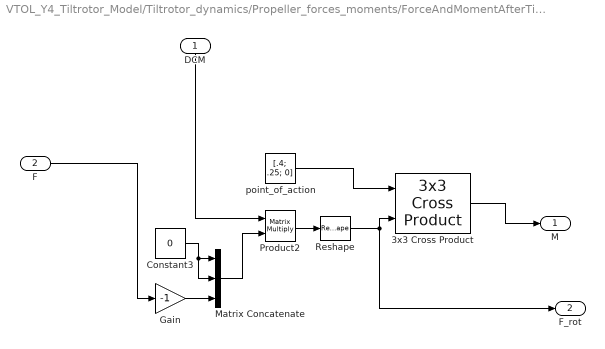
== system VTOL_Y4_Tiltrotor_Model/Tiltrotor_dynamics/Propeller_forces_moments/ForceAndMomentAfterTilting1 ==
  DCM : Inport
  F : Inport  Port=2
  3x3 Cross Product : aerolibutil/3x3 Cross Product
  Constant3 : Constant  Value=0
  Gain : Gain  Gain=-1
  Matrix Concatenate : Concatenate  NumInputs=3  ConcatenateDimension=2
  Product2 : Product  Multiplication=Matrix(*)
  Reshape : Reshape  OutputDimensionality=Customize  OutputDimensions=[3,1]
  point_of_action : Constant  Value="[.4;  .25;  0]"  VectorParams1D=off
  M : Outport
  F_rot : Outport  Port=2
  wires:
  Reshape/1 -> F_rot/1, 3x3 Cross Product/2
  Product2/1 -> Reshape/1
  point_of_action/1 -> 3x3 Cross Product/1
  Constant3/1 -> Matrix Concatenate/1, Matrix Concatenate/2
  Matrix Concatenate/1 -> Product2/2
  DCM/1 -> Product2/1
  F/1 -> Gain/1
  3x3 Cross Product/1 -> M/1
  Gain/1 -> Matrix Concatenate/3

== system VTOL_Y4_Tiltrotor_Model/Tiltrotor_dynamics/Propeller_forces_moments/ForceAndMomentAfterTilting2 ==
  DCM : Inport
  F : Inport  Port=2
  3x3 Cross Product : aerolibutil/3x3 Cross Product
  Constant3 : Constant  Value=0
  Gain : Gain  Gain=-1
  Matrix Concatenate : Concatenate  NumInputs=3  ConcatenateDimension=2
  Product2 : Product  Multiplication=Matrix(*)
  Reshape : Reshape  OutputDimensionality=Customize  OutputDimensions=[3,1]
  point_of_action : Constant  Value="[-.4;  0;  0]"  VectorParams1D=off
  M : Outport
  F_rot : Outport  Port=2
  wires:
  3x3 Cross Product/1 -> M/1
  F/1 -> Gain/1
  DCM/1 -> Product2/1
  Matrix Concatenate/1 -> Product2/2
  Constant3/1 -> Matrix Concatenate/2, Matrix Concatenate/1
  point_of_action/1 -> 3x3 Cross Product/1
  Product2/1 -> Reshape/1
  Reshape/1 -> 3x3 Cross Product/2, F_rot/1
  Gain/1 -> Matrix Concatenate/3

== system VTOL_Y4_Tiltrotor_Model/Tiltrotor_dynamics/Propeller_forces_moments/ForceAndMomentAfterTilting3 ==
  DCM : Inport
  F : Inport  Port=2
  3x3 Cross Product : aerolibutil/3x3 Cross Product
  Constant3 : Constant  Value=0
  Gain : Gain  Gain=-1
  Matrix Concatenate : Concatenate  NumInputs=3  ConcatenateDimension=2
  Product2 : Product  Multiplication=Matrix(*)
  Reshape : Reshape  OutputDimensionality=Customize  OutputDimensions=[3,1]
  point_of_action : Constant  Value="[-.4;  0;  0]"  VectorParams1D=off
  M : Outport
  F_rot : Outport  Port=2
  wires:
  Reshape/1 -> F_rot/1, 3x3 Cross Product/2
  Product2/1 -> Reshape/1
  point_of_action/1 -> 3x3 Cross Product/1
  Constant3/1 -> Matrix Concatenate/1, Matrix Concatenate/2
  Matrix Concatenate/1 -> Product2/2
  DCM/1 -> Product2/1
  F/1 -> Gain/1
  3x3 Cross Product/1 -> M/1
  Gain/1 -> Matrix Concatenate/3
